simulink model "EKF_03"  (R2015a)
settings: Solver=ode45  StartTime=0.0  StopTime=40  RelTol=1e-3
model workspace: external: MAT-File Init_Model_02_Simulink.mat (data not in the file)
values from neighbouring files (symbols this model uses):
  Cov_nu = [0.005 0 0 0 ... (first row only)    [InitOOSM.m]    (also in InitSIL.m; Init_Model_02_Simulink.m; Init_Model_02_Simulink_SIL1.m)
  Cov_r = [0.003 0 0 ... (first row only)    [InitOOSM.m]    (also in InitSIL.m; Init_Model_02_Simulink.m; Init_Model_02_Simulink_SIL1.m)
  e_force_x = 0    [InitOOSM.m]    (also in InitSIL.m; Init_Model_02_Simulink.m; Init_Model_02_Simulink_SIL1.m)
  e_force_y = 0    [InitOOSM.m]    (also in InitSIL.m; Init_Model_02_Simulink.m; Init_Model_02_Simulink_SIL1.m)
  e_force_z = 0    [InitOOSM.m]    (also in InitSIL.m; Init_Model_02_Simulink.m; Init_Model_02_Simulink_SIL1.m)
  ita = [0.5;0.5;0.5;0.5]    [InitOOSM.m]    (also in InitSIL.m; Init_Model_02_Simulink.m = [0.12; 0.05; -0.15; 0.98]; Init_Model_02_Simulink_SIL1.m)
  n = 0.00    (= 0)    [InitOOSM.m]    (also in InitSIL.m; Init_Model_02_Simulink.m = 0.0012; Init_Model_02_Simulink_SIL1.m)
  P_d = Simulink.Signal    [InitOOSM.m]    (also in InitSIL.m; Init_Model_02_Simulink.m; Init_Model_02_Simulink_SIL1.m)
  P_k = Simulink.Signal    [InitOOSM.m]    (also in InitSIL.m; Init_Model_02_Simulink.m; Init_Model_02_Simulink_SIL1.m)
  p_x = 0.75    [InitOOSM.m]    (also in InitSIL.m; Init_Model_02_Simulink.m; Init_Model_02_Simulink_SIL1.m)
  p_y = 0.125    [InitOOSM.m]    (also in InitSIL.m; Init_Model_02_Simulink.m; Init_Model_02_Simulink_SIL1.m)
  p_z = -0.8    [InitOOSM.m]    (also in InitSIL.m; Init_Model_02_Simulink.m; Init_Model_02_Simulink_SIL1.m)
  parameter_gravitation = 3.986005E+14    (= 398600500000000)    [InitOOSM.m]    (also in InitSIL.m; Init_Model_02_Simulink.m; Init_Model_02_Simulink_SIL1.m)
  rho = [0.04;0;0.3]    [InitOOSM.m]    (also in InitSIL.m; Init_Model_02_Simulink.m = [0.2; 0.1; 0.05]; Init_Model_02_Simulink_SIL1.m)
  rho_c = [-0.00017;   -0.9780;   -0.1854]    [InitOOSM.m]    (also in InitSIL.m = [0.00036;   -0.9865;   -0.1854]; Init_Model_02_Simulink.m = [0; 0; 0.9]; Init_Model_02_Simulink_SIL1.m = [0.00036;   -0.9865;   -0.1854])
  sig_f = 2E-6    (= 2e-06)    [InitOOSM.m]    (also in InitSIL.m; Init_Model_02_Simulink.m; Init_Model_02_Simulink_SIL1.m)
  sig_tau = 2.5E-5    (= 2.5e-05)    [InitOOSM.m]    (also in InitSIL.m; Init_Model_02_Simulink.m; Init_Model_02_Simulink_SIL1.m)
  t_delta = 0.2    [InitOOSM.m]    (also in InitSIL.m; Init_Model_02_Simulink.m = 0.1; Init_Model_02_Simulink_SIL1.m)
  t_Kalman = 0.01    [InitOOSM.m]    (also in InitSIL.m; Init_Model_02_Simulink.m; Init_Model_02_Simulink_SIL1.m)
  t_Sim = 0.001    [InitOOSM.m]    (also in InitSIL.m; Init_Model_02_Simulink.m; Init_Model_02_Simulink_SIL1.m)
  tau_1 = 0    [InitOOSM.m]    (also in InitSIL.m; Init_Model_02_Simulink.m; Init_Model_02_Simulink_SIL1.m)
  tau_2 = 0    [InitOOSM.m]    (also in InitSIL.m; Init_Model_02_Simulink.m; Init_Model_02_Simulink_SIL1.m)
  tau_3 = 0    [InitOOSM.m]    (also in InitSIL.m; Init_Model_02_Simulink.m; Init_Model_02_Simulink_SIL1.m)
  U_n_d = Simulink.Signal    [InitOOSM.m]    (also in InitSIL.m; Init_Model_02_Simulink.m; Init_Model_02_Simulink_SIL1.m)
  X_a_0 = [0; 0; 0; 1; 0; 0; 0; 0; 0; 0; 0; 0; 0;0;0;0;0;0;0;1]    [InitOOSM.m]    (also in InitSIL.m = [0; 0; 0; 1; 0; 0; 0; 0; 0; 0; 0; 0; 0]; Init_Model_02_Simulink.m = [0; 0; 0; 1; 0; 0; 0; 0; 0; 0; 0; 0; 0]; Init_Model_02_Simulink_SIL1.m = [0;0;0.707;0.707;0.2;-0.02;0.0001;0.02;-1.80;0.50;-0.05;0.00)
  x_d = Simulink.Signal    [InitOOSM.m]    (also in InitSIL.m; Init_Model_02_Simulink.m; Init_Model_02_Simulink_SIL1.m)
  x_k = Simulink.Signal    [InitOOSM.m]    (also in InitSIL.m; Init_Model_02_Simulink.m; Init_Model_02_Simulink_SIL1.m)
undefined symbols (not defined in the file or in its folder): des, gcbh
libraries: simulink x5, dspmtrx3 x1
(part 5 of 5)

== matlab function EKF_03/OOSM_KF/OOSM_KF/State Propagation1/MATLAB Function ==
  data: X_a input; Phi output; n input; t_Kalman input; p input; M input
%Function: fn_Create_Phi()
%Inputs: X_a - 23-state vector,
%        n - angular velocity of spacecrafts,
%        t_delta - sampling time
%Outputs: [Phi] (State-propagation Matrix)
%Functionality: Generates the State Propagation matrix
%Author: Hrishik Mishra
function Phi  = fn_Create_Phi(X_a,n,t_Kalman,p,M)
    Phi_t = fn_Create_Phi_t(n,t_Kalman);
    Phi_r = fn_Create_Phi_r(X_a,p, t_Kalman);
    Phi = [Phi_r, zeros(6,6);zeros(6,6),Phi_t];

end
%Create state propagation matrix of the whole system

%Function: fn_Create_Phi_r()
%Inputs: X_a - 23-state vector,
%Outputs: [Phi_r] (State-propagation Matrix for Rotation component)
%Functionality: Generates the State Propagation matrix for Rotation
%component
%Author: Hrishik Mishra
function [Phi_r] = fn_Create_Phi_r(X_a,p,t_Kalman) 
    Phi_r = zeros(6,6);
    omega = X_a(5:7);
    M = fn_Create_M(p,omega);   
    
    A = [-fn_VectorToSkewSymmetricTensor(omega),0.5*eye(3,3);zeros(3,3),M];
    Phi_r = expm(A*t_Kalman);
%     phi_r11 = fn_Create_phi_r11(omega,t_delta);
%     phi_r12 = fn_Create_phi_r12(omega,M,t_delta);
%     phi_r22 = fn_Create_phi_r22(omega,t_delta,M);
%     phi_r13 = fn_Create_phi_r13(omega,t_delta,M,N);
%     phi_r23 = fn_Create_phi_r23(omega,t_delta,M,N);
%     Phi_r = [phi_r11, phi_r12, phi_r13;zeros(3,3),phi_r22,phi_r23;zeros(3,3),zeros(3,3),eye(3,3)];
%     

end
%Function: fn_Create_M()
%Inputs: p - Inertial ratios 
%        omega - angular velocity between Chaser Grasping frame and Chaser
%        CoM
%Outputs: M (Linearized model matrix for inertial parameters)
%Functionality: Generates M
%Author: Hrishik Mishra
function M = fn_Create_M(p,omega)
    %#Codegen
    
    M = [0, p(1)*omega(3), p(1)*omega(2); p(2)*omega(3), 0, p(2)*omega(1); p(3)*omega(2),p(3)*omega(1),0];
end
%Function: fn_Create_N()
%Inputs: omega - angular velocity between Chaser Grasping frame and Chaser
%        CoM
%Outputs: N (Linearized model matrix for inertial parameters)
%Functionality: Generates M
%Author: Hrishik Mishra
function N = fn_Create_N(omega)
%
    N = [omega(2)*omega(3), 0, 0; 0, omega(1)*omega(3), 0; 0, 0, omega(1)*omega(2)];
end

%%
%Function: fn_Create_Phi_t()
%Inputs: n - angular velocity of Chaser/Target (almost same)
%        t_delta - sampling time
%Outputs: Phi_t (State Transition Matrix for Translation component)
%Functionality: Generates Phi_t
%Author: Hrishik Mishra
function Phi_t = fn_Create_Phi_t(n,t_delta)
%
    Phi_t12 = [t_delta, n*t_delta^2,0;0, t_delta, 0;0,0,t_delta];
    Phi_t22 = eye(3,3) - 2*fn_VectorToSkewSymmetricTensor([0;0;n])*t_delta;
    
    Phi_t = [eye(3,3),Phi_t12;zeros(3,3),Phi_t22];
    
end

== matlab function EKF_03/EKF/Measurement Update/Compute_K_d/Measurement noise covariance ==
  data: q_nominal input; S output; ita_nominal input; cov_r input; cov_nu input
%Function: fn_Create_S()
%Inputs: q_nominal: Quaternion between Chaser CoM and Target CoM
%        ita_nominal: Quaternion between Target CoM and Target grasping
%        frame
%        cov_r: position covariance due to camera
%        cov_nu: orientation covariance due to camera
%Outputs: S (Measurement noise covariance Matrix)
%Functionality: Generates S
%Author: Hrishik Mishra
function S   = fn_Create_S(q_nominal,ita_nominal,cov_r,cov_nu)
    %#codegen
    q_star = [-q_nominal(1:3);q_nominal(4)];
    ita_star = [-ita_nominal(1:3);ita_nominal(4)];
    Ita_Tensor = fn_CrossTensor(ita_star,0);
    Q_Tensor = fn_CrossTensor(q_star,1);
    T = [eye(3,3),zeros(3,1)]*Ita_Tensor*Q_Tensor;
    S = [cov_r,zeros(3,3);zeros(3,3), T*cov_nu*T'];
end

== matlab function EKF_03/EKF/Measurement Update/Create h_d/Subsystem/MATLAB Function2 ==
  data: q input; CrossTensor output; flag input
%Inputs: q: quaternion vector
%        flag:0-cross;1-star
function CrossTensor  = fn_CrossTensor(q,flag)
    %#codegen
    CrossTensor = zeros(4,4);
    q_v = q(1:3);
    q_0 = q(4);    
    cross_q_v = fn_VectorToSkewSymmetricTensor(q_v);
    switch (flag)
        case 0
            CrossTensor = [-cross_q_v + q_0*eye(3,3), q_v;-q_v',q_0];
        case 1
            CrossTensor = [cross_q_v + q_0*eye(3,3), q_v;-q_v',q_0];
        otherwise
            
    end
end

== matlab function EKF_03/EKF/Measurement Update/Propagate_state (full)/Create q_nominal/Create nominal q/MATLAB Function ==
  data: q input; CrossTensor output; flag input
%Inputs: q: quaternion vector
%        flag:0-cross;1-star
function CrossTensor  = fn_CrossTensor(q,flag)
    %#codegen
    CrossTensor = zeros(4,4);
    q_v = q(1:3);
    q_0 = q(4);    
    cross_q_v = fn_VectorToSkewSymmetricTensor(q_v);
    switch (flag)
        case 0
            CrossTensor = [-cross_q_v + q_0*eye(3,3), q_v;-q_v',q_0];
        case 1
            CrossTensor = [cross_q_v + q_0*eye(3,3), q_v;-q_v',q_0];
        otherwise
            
    end
end

== matlab function EKF_03/EKF/Measurement Update/Propagate_state (full)/Create q_nominal/Create nominal q/MATLAB Function1 ==
  data: A input; exponent_A output
function exponent_A = fcn(A)
%#codegen
    exponent_A = expm(A);
end

== matlab function EKF_03/EKF/Predictor/Dynamic Model (Differential equations)1/Dynamic Model (Differential equations)/Quaternion Kinematics/MATLAB Function ==
  data: q input; CrossTensor output; flag input
%Inputs: q: quaternion vector
%        flag:0-cross;1-star
function CrossTensor  = fn_CrossTensor(q,flag)
    %#codegen
    CrossTensor = zeros(4,4);
    q_v = q(1:3);
    q_0 = q(4);    
    cross_q_v = fn_VectorToSkewSymmetricTensor(q_v);
    switch (flag)
        case 0
            CrossTensor = [-cross_q_v + q_0*eye(3,3), q_v;-q_v',q_0];
        case 1
            CrossTensor = [cross_q_v + q_0*eye(3,3), q_v;-q_v',q_0];
        otherwise
            
    end
end

== matlab function EKF_03/EKF/Measurement Update/Propagate_state (full)/State Propagation1/MATLAB Function ==
  data: X_a input; Phi output; n input; t_Kalman input; p input; M input
%Function: fn_Create_Phi()
%Inputs: X_a - 23-state vector,
%        n - angular velocity of spacecrafts,
%        t_delta - sampling time
%Outputs: [Phi] (State-propagation Matrix)
%Functionality: Generates the State Propagation matrix
%Author: Hrishik Mishra
function Phi  = fn_Create_Phi(X_a,n,t_Kalman,p,M)
    Phi_t = fn_Create_Phi_t(n,t_Kalman);
    Phi_r = fn_Create_Phi_r(X_a,p, t_Kalman);
    Phi = [Phi_r, zeros(6,6);zeros(6,6),Phi_t];

end
%Create state propagation matrix of the whole system

%Function: fn_Create_Phi_r()
%Inputs: X_a - 23-state vector,
%Outputs: [Phi_r] (State-propagation Matrix for Rotation component)
%Functionality: Generates the State Propagation matrix for Rotation
%component
%Author: Hrishik Mishra
function [Phi_r] = fn_Create_Phi_r(X_a,p,t_Kalman) 
    Phi_r = zeros(6,6);
    omega = X_a(5:7);
    M = fn_Create_M(p,omega);   
    
    A = [-fn_VectorToSkewSymmetricTensor(omega),0.5*eye(3,3);zeros(3,3),M];
    Phi_r = expm(A*t_Kalman);
%     phi_r11 = fn_Create_phi_r11(omega,t_delta);
%     phi_r12 = fn_Create_phi_r12(omega,M,t_delta);
%     phi_r22 = fn_Create_phi_r22(omega,t_delta,M);
%     phi_r13 = fn_Create_phi_r13(omega,t_delta,M,N);
%     phi_r23 = fn_Create_phi_r23(omega,t_delta,M,N);
%     Phi_r = [phi_r11, phi_r12, phi_r13;zeros(3,3),phi_r22,phi_r23;zeros(3,3),zeros(3,3),eye(3,3)];
%     

end
%Function: fn_Create_M()
%Inputs: p - Inertial ratios 
%        omega - angular velocity between Chaser Grasping frame and Chaser
%        CoM
%Outputs: M (Linearized model matrix for inertial parameters)
%Functionality: Generates M
%Author: Hrishik Mishra
function M = fn_Create_M(p,omega)
    %#Codegen
    
    M = [0, p(1)*omega(3), p(1)*omega(2); p(2)*omega(3), 0, p(2)*omega(1); p(3)*omega(2),p(3)*omega(1),0];
end
%Function: fn_Create_N()
%Inputs: omega - angular velocity between Chaser Grasping frame and Chaser
%        CoM
%Outputs: N (Linearized model matrix for inertial parameters)
%Functionality: Generates M
%Author: Hrishik Mishra
function N = fn_Create_N(omega)
%
    N = [omega(2)*omega(3), 0, 0; 0, omega(1)*omega(3), 0; 0, 0, omega(1)*omega(2)];
end

%%
%Function: fn_Create_Phi_t()
%Inputs: n - angular velocity of Chaser/Target (almost same)
%        t_delta - sampling time
%Outputs: Phi_t (State Transition Matrix for Translation component)
%Functionality: Generates Phi_t
%Author: Hrishik Mishra
function Phi_t = fn_Create_Phi_t(n,t_delta)
%
    Phi_t12 = [t_delta, n*t_delta^2,0;0, t_delta, 0;0,0,t_delta];
    Phi_t22 = eye(3,3) - 2*fn_VectorToSkewSymmetricTensor([0;0;n])*t_delta;
    
    Phi_t = [eye(3,3),Phi_t12;zeros(3,3),Phi_t22];
    
end
